simulink model "LW_ctrl"  (R2024b)
settings: Solver=ode4  StartTime=0.0  StopTime=SIM_TIME  FixedStep=0.001  RelTol=1e-3  EnableMultiTasking=on
StartFcn:
  | %timestart = cputime;
StopFcn:
  | %dt = cputime - timestart
undefined symbols (not defined in the file or in its folder): AttCtrl_cycle, ControlMode, DEG2RAD, Earth, FlightMode, LW_ACRO_P_MAX, LW_ACRO_R_MAX, LW_ACRO_Y_MAX, LW_AERO_C0, LW_AERO_C1, LW_AERO_Y0, LW_ANGLE, LW_DMZ0, LW_DMZ_MIN, LW_LAT_CIRCLE, LW_MAN_PITCH_MAX, LW_MAN_ROLL_MAX, LW_MASS, LW_OB_CIRCLE_R, LW_OB_CIRCLE_V, LW_OB_CIRCLE_W, LW_OB_TYPE, LW_REX_YAW, LW_SERVOL_MAX, LW_SERVOR_MAX, LW_THR_HOVER, LW_WZ_MAX, LW_X_ACCEL_MAX, LW_X_ACCEL_MIN, LW_X_FF, LW_X_JERK_MAX, LW_X_P, LW_X_VEL_MAX, LW_Y_ACCEL_MAX, LW_Y_ACCEL_MIN, LW_Y_FF, LW_Y_JERK_MAX, LW_Y_P, LW_Y_VEL_MAX, LW_YAW_KAD, LW_YAW_KAP, LW_Z_ACCEL_LOW, LW_Z_ACCEL_UP, LW_Z_FF, LW_Z_JERK_MAX, LW_Z_P, LW_Z_VEL_MAX_UP, Map_xoffset, Map_yoffset, Map_zoffset, MAX_wdotx, MAX_wdoty, MAX_wdotz, Mixer_cycle, ModelParam_AccelMax, ModelParam_DelayAtt, ModelParam_DelayOmega, ModelParam_DelayPos, ModelParam_envAltitude, ModelParam_envGravityAcc ... (+57)
libraries: pixhawk_slib_uORB_RW x15, simulink x6, slpidlib x6, dspstat3 x5, aerolibnav x4, aerolibtransform2 x3, pixhawk_slib_sensors_actuators x2, etargetslib x2, pixhawk_slib_rfly x1, aerolibatmos2 x1, slrealtimeiplib x1, SignalEditorBlockLib x1
(part 3 of 6)

== system LW_ctrl/Controller/PID_Controller/PID_Controller/toPWM ==
  T : Inport
  voltage : Inport  Port=2
  Bus Selector2 : BusSelector  OutputSignals=battery_status.voltage_filtered_v,battery_status.connected
  Constant : Constant  Value=single(1/ModelParam_rotorCt)
  Product : Product
  Sqrt : Sqrt
  toPWM : MATLAB Function  TreatAsAtomicUnit=on
  pwm : Outport  VectorParamsAs1DForOutWhenUnconnected=off
  wires:
  T/1 -> Product/1
  Product/1 -> Sqrt/1
  toPWM/1(pwm) -> pwm/1
  Constant/1 -> Product/2
  Sqrt/1 -> toPWM/1(w)
  voltage/1 -> Bus Selector2/1
  Bus Selector2/1 -> toPWM/2(voltage)  "<voltage_filtered_v>"
  Bus Selector2/2 -> toPWM/3(batt_connected)  "<connected>"

== system LW_ctrl/Output/OutputSelect/Sim/Lifting Body Airframe ==
  inPWM : Inport
  Constant : Constant  Value=SEND_TO_UNREAL
  Constant1 : Constant  Value=0
  Constant2 : Constant  Value=[0 0 0 0 0 0]  OutDataTypeStr=single
  Estimator : Subsystem
  Get Terrain : Subsystem
  Selector : Selector  InputPortWidth=8  IndexOptions=Index vector (dialog)  Indices=[1:6]  OutputSizes=1
  Subsystem Reference : Subsystem  ReferencedSubsystem=LW_noaileron_dynamic
  Switch : Switch  Criteria=u2 ~= 0  SaturateOnIntegerOverflow=off  InputSameDT=off
  Terminator : Terminator
  To Unreal : Subsystem  InitFcn=RflySim3D_config
  wires:
  inPWM/1 -> Selector/1
  Subsystem Reference/1 -> Estimator/1(vehicle_states), Get Terrain/1(vehicle_states), To Unreal/1(vehicle_states)  "vehicle_sates"
  Subsystem Reference/2 -> Estimator/2(environment_states)  "env_states"
  Subsystem Reference/3 -> Terminator/1
  Subsystem Reference/4 -> To Unreal/2(MotorRads)
  Get Terrain/1(z) -> Switch/1
  Constant/1 -> Switch/2
  Switch/1 -> Subsystem Reference/2
  Constant1/1 -> Switch/3
  Selector/1 -> Subsystem Reference/1  "pwm1~6"
  Constant2/1 -> Subsystem Reference/3

== system LW_ctrl/navigator/logger/HIL&FLY/get_delta_t ==
  timestamp : Inport
  Data Type Conversion : DataTypeConversion  OutDataTypeStr=single  SaturateOnIntegerOverflow=off  RndMeth=Floor
  Gain : Gain  Gain=1.0e-6
  Memory : Memory  InheritSampleTime=on
  Saturation : Saturate  UpperLimit=0.2  LowerLimit=0.001
  Sum : Sum  Inputs=|+-
  delta_t : Outport  VectorParamsAs1DForOutWhenUnconnected=off
  wires:
  Gain/1 -> Saturation/1
  timestamp/1 -> Memory/1, Sum/1
  Memory/1 -> Sum/2
  Sum/1 -> Gain/1
  Data Type Conversion/1 -> delta_t/1
  Saturation/1 -> Data Type Conversion/1

== system LW_ctrl/navigator/navigator_offboard/task select/task select ==
  timestamp : Inport
  flight_mode : Inport  Port=2
  pos : Inport  Port=3
  vel : Inport  Port=4
  q : Inport  Port=5
  v_wind : Inport  Port=6
  CH8 : Inport  Port=7
  Bus Creator2 : BusCreator  Inputs=10  OutDataTypeStr=Bus: offboard_bus
      settings: InheritFromInputs=off
  df,coor,wind : MATLAB Function  TreatAsAtomicUnit=on
  task : MATLAB Function  TreatAsAtomicUnit=on
  task1 : Outport
  wires:
  df,coor,wind/3(acc_ref) -> Bus Creator2/3  "acc"
  df,coor,wind/10(OB_TASK) -> Bus Creator2/10
  task/4(euler_ref) -> df,coor,wind/4(euler_ref)
  task/7(dotpsi) -> df,coor,wind/7(dotpsi)
  task/5(dot3x) -> df,coor,wind/5(dot3x)
  df,coor,wind/1(pos_ref) -> Bus Creator2/1  "pos"
  Bus Creator2/1 -> task1/1
  df,coor,wind/9(dotwb_ref) -> Bus Creator2/9
  df,coor,wind/7(beta) -> Bus Creator2/7
  flight_mode/1 -> task/2(flight_mode)
  df,coor,wind/2(vel_ref) -> Bus Creator2/2  "vel"
  task/3(acc_ref) -> df,coor,wind/3("acc_ref ")
  task/1(pos_ref) -> df,coor,wind/1("pos_ref ")
  task/2(vel_ref) -> df,coor,wind/2("vel_ref ")
  task/6(yaw_ref) -> df,coor,wind/6(yaw_ref)
  df,coor,wind/5(f_d) -> Bus Creator2/5
  df,coor,wind/8(wb_ref) -> Bus Creator2/8
  q/1 -> task/5(q)
  df,coor,wind/6(alpha) -> Bus Creator2/6
  df,coor,wind/4(q_ref) -> Bus Creator2/4  "q"
  timestamp/1 -> task/1(timestamp)
  pos/1 -> task/3(pos)
  vel/1 -> task/4(vel)
  v_wind/1 -> df,coor,wind/8(v_wind)
  CH8/1 -> task/6(CH8)

== system LW_ctrl/rc_receive/manual_ctrl_in/HIL&FLY V1.13.3/logger ==
  Bus Selector : BusSelector  OutputSignals=x,y,r,z,AU5,AU6,AU7,AU8,RC_Lost
  Data Type Conversion : DataTypeConversion  Priority=10  OutDataTypeStr=double  SaturateOnIntegerOverflow=off  RndMeth=Floor
  Data Type Conversion{1..4} (4 alike) : DataTypeConversion  Priority=10  OutDataTypeStr=single  SaturateOnIntegerOverflow=off  RndMeth=Floor
  Data Type Conversion{5..7,9} (4 alike) : DataTypeConversion  Priority=10  OutDataTypeStr=uint32  SaturateOnIntegerOverflow=off  RndMeth=Floor
  Data Type Conversion8 : DataTypeConversion  Priority=10  OutDataTypeStr=boolean  SaturateOnIntegerOverflow=off  RndMeth=Floor
  get_delta_t : Subsystem
  hrt_timestamp : MATLAB Function  TreatAsAtomicUnit=on
  uORB Write Advanced : pixhawk_slib_uORB_RW/uORB Write Advanced  Ts=0  uORB_AdvtQueue=on  uORB_FieldEnabledArr="0  0  0  1  0  0  0  0  0  0  0"  uORB_Topic_str=0  uORB_Struct_DT="[1  1  1  1  1]"  BlockInputCount=5  uORB_StructParams="[\"voltage_v\",\"voltage_filtered_v\",\"current_a\",\"current_filtered_a\",\"remaining\"]"  uORB_PortSizes="[1  1  1  1]"  MsgSizeOf=0  MW_update=true
      settings: SourceProductName=uORB Read / Write Blocks
  wires:
  hrt_timestamp/1(ts) -> Data Type Conversion/1
  Data Type Conversion/1 -> uORB Write Advanced/1, get_delta_t/1(timestamp)
  get_delta_t/1(delta_t) -> uORB Write Advanced/2
  [log_man] -> Bus Selector/1  "log_man"
  Bus Selector/1 -> Data Type Conversion1/1  "<x>"
  Bus Selector/2 -> Data Type Conversion2/1  "<y>"
  Bus Selector/3 -> Data Type Conversion3/1  "<r>"
  Bus Selector/4 -> Data Type Conversion4/1  "<z>"
  Bus Selector/5 -> Data Type Conversion5/1  "<AU5>"
  Bus Selector/6 -> Data Type Conversion6/1  "<AU6>"
  Bus Selector/7 -> Data Type Conversion7/1  "<AU7>"
  Bus Selector/9 -> Data Type Conversion8/1  "<RC_Lost>"
  Data Type Conversion1/1 -> uORB Write Advanced/3
  Data Type Conversion2/1 -> uORB Write Advanced/4
  Data Type Conversion3/1 -> uORB Write Advanced/5
  Data Type Conversion4/1 -> uORB Write Advanced/6
  Data Type Conversion5/1 -> uORB Write Advanced/7
  Data Type Conversion6/1 -> uORB Write Advanced/8
  Data Type Conversion7/1 -> uORB Write Advanced/9
  Data Type Conversion8/1 -> uORB Write Advanced/11
  Bus Selector/8 -> Data Type Conversion9/1  "<AU8>"
  Data Type Conversion9/1 -> uORB Write Advanced/10

== system LW_ctrl/rc_receive/manual_ctrl_in/Sim/Simulate RC ==
  Bus Creator : BusCreator  Inputs=9
  CH1 : Constant  Value=1500  OutDataTypeStr=uint16
  CH2 : Constant  Value=1500  OutDataTypeStr=uint16
  CH3 : Constant  Value=1600  OutDataTypeStr=uint16
  CH4 : Constant  Value=1500  OutDataTypeStr=uint16
  CH5 : Constant  Value=1000  OutDataTypeStr=uint16
  CH6 : Constant  Value=1000  OutDataTypeStr=uint16  SampleTime=-1
  CH7 : Constant  Value=1000  OutDataTypeStr=uint16
  CH8 : Constant  Value=1000  OutDataTypeStr=uint16
  Data Type Conversion{,1..4} (5 alike) : DataTypeConversion  OutDataTypeStr=single  SaturateOnIntegerOverflow=off  RndMeth=Floor
  InputConditioning : Subsystem
  RC_LOST : Constant  Value=false  OutDataTypeStr=uint16
  manual_ctrl_in : Outport  VectorParamsAs1DForOutWhenUnconnected=off
  wires:
  CH7/1 -> Data Type Conversion3/1
  Data Type Conversion1/1 -> Bus Creator/6  "AU6"
  InputConditioning/1(x) -> Bus Creator/1  "x"
  Bus Creator/1 -> manual_ctrl_in/1
  CH1/1 -> InputConditioning/1("ch1 ")
  InputConditioning/3(r) -> Bus Creator/3  "r"
  CH4/1 -> InputConditioning/4(ch4)
  InputConditioning/4(z) -> Bus Creator/4  "z"
  InputConditioning/2(y) -> Bus Creator/2  "y"
  Data Type Conversion3/1 -> Bus Creator/7  "AU7"
  Data Type Conversion/1 -> Bus Creator/5  "AU5"
  Data Type Conversion2/1 -> Bus Creator/9  "RC_Lost"
  CH2/1 -> InputConditioning/2(ch2)
  CH5/1 -> Data Type Conversion/1
  RC_LOST/1 -> Data Type Conversion2/1
  CH3/1 -> InputConditioning/3(ch3)
  CH6/1 -> Data Type Conversion1/1
  Data Type Conversion4/1 -> Bus Creator/8  "AU8"
  CH8/1 -> Data Type Conversion4/1

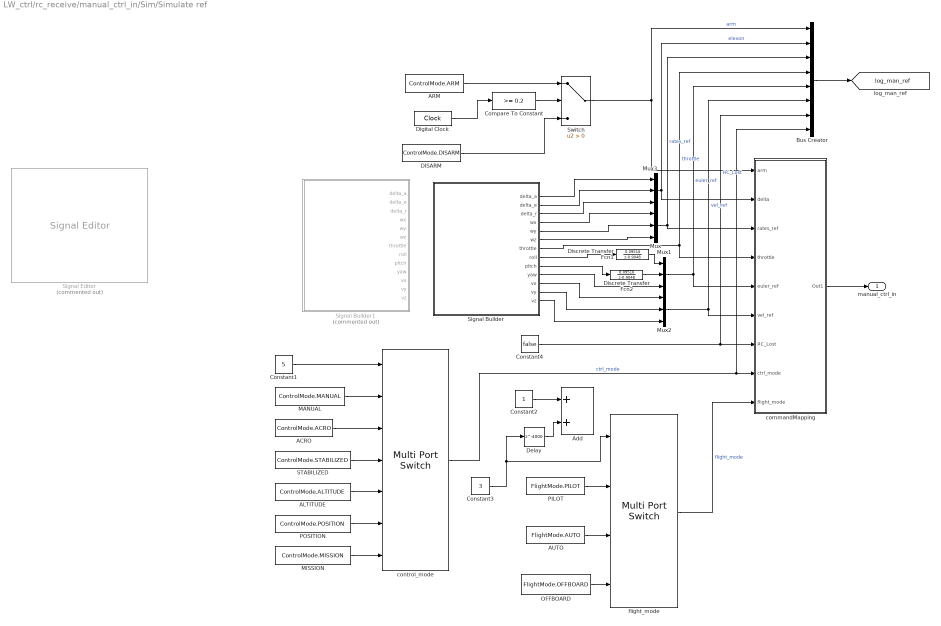
== system LW_ctrl/rc_receive/manual_ctrl_in/Sim/Simulate ref ==
  ACRO : Constant  Value=ControlMode.ACRO
  ALTITUDE : Constant  Value=ControlMode.ALTITUDE
  ARM : Constant  Value=ControlMode.ARM
  AUTO : Constant  Value=FlightMode.AUTO
  Add : Sum
  Bus Creator : BusCreator  Inputs=8
  Compare To Constant : simulink/Logic and Bit Operations/Compare To Constant  relop=>=  const=0.2  OutDataTypeStr=boolean
  Constant1 : Constant  Value=5
  Constant2 : Constant
  Constant3 : Constant  Value=3
  Constant4 : Constant  Value=false
  DISARM : Constant  Value=ControlMode.DISARM
  Delay : Delay  DelayLength=4000  InitialCondition=0
  Digital Clock : DigitalClock  SampleTime=-1
  Discrete Transfer Fcn1 : DiscreteTransferFcn  Numerator=0.09516  Denominator=[1 -0.9048]
  Discrete Transfer Fcn2 : DiscreteTransferFcn  Numerator=0.09516  Denominator=[1 -0.9048]
  MANUAL : Constant  Value=ControlMode.MANUAL
  MISSION : Constant  Value=ControlMode.MISSION
  Mux{,1..3} (4 alike) : Mux  Inputs=3
  OFFBOARD : Constant  Value=FlightMode.OFFBOARD
  PILOT : Constant  Value=FlightMode.PILOT
  POSITION : Constant  Value=ControlMode.POSITION
  STABILIZED : Constant  Value=ControlMode.STABILIZED
  Signal Builder : Subsystem  Tag=STV Subsys  LoadFcn=sigbuilder_block('load');  StartFcn=sigbuilder_block('start');  StopFcn=sigbuilder_block('stop');  ClipboardFcn=sigbuilder_block('clipboard');  TreatAsAtomicUnit=on  mask(Sigbuilder block){tuvar=[0:10]}
      mask help: Simulink:masks:SigbuilderBlock_MD
      mask init:
      | if ~strcmp(get_param(bdroot(gcbh),'SimulationStatus'),'stopped') tuvar = sigbuilder_block('maskInit'); end
      settings: CopyFcn=sigbuilder_block('copy');  DeleteFcn=sigbuilder_block('delete');  ModelCloseFcn=sigbuilder_block('modelClose');  PreSaveFcn=sigbuilder_block('preSave');  PauseFcn=sigbuilder_block('pause');  ContinueFcn=sigbuilder_block('continue');  NameChangeFcn=sigbuilder_block('namechange');  OpenFcn=sigbuilder_block('open',[16 10 1269 593 ]);  CloseFcn=sigbuilder_block('close');
      mask Display: plot(0, 0, 100, 100,[2, 2, 32, 32, 2], [68, 8, 8, 68, 68],[32, 2], [38, 38], [32, 19, 2],[53, 60, 44], [32, 17, 17, 2],[16, 16, 31, 31]);txt = getActiveGroup(gcbh);text(2, 100, txt,'verticalAlignment', 'top');
  Signal Builder1 : Subsystem  Tag=STV Subsys  Commented=on  LoadFcn=sigbuilder_block('load');  StartFcn=sigbuilder_block('start');  StopFcn=sigbuilder_block('stop');  ClipboardFcn=sigbuilder_block('clipboard');  TreatAsAtomicUnit=on  mask(Sigbuilder block){tuvar=[0:10]}
      mask help: Simulink:masks:SigbuilderBlock_MD
      mask init:
      | if ~strcmp(get_param(bdroot(gcbh),'SimulationStatus'),'stopped') tuvar = sigbuilder_block('maskInit'); end
      settings: CopyFcn=sigbuilder_block('copy');  DeleteFcn=sigbuilder_block('delete');  ModelCloseFcn=sigbuilder_block('modelClose');  PreSaveFcn=sigbuilder_block('preSave');  PauseFcn=sigbuilder_block('pause');  ContinueFcn=sigbuilder_block('continue');  NameChangeFcn=sigbuilder_block('namechange');  OpenFcn=sigbuilder_block('open',[0 0 1380.75 751.5 ]);  CloseFcn=sigbuilder_block('close');
      mask Display: plot(0, 0, 100, 100,[2, 2, 32, 32, 2], [68, 8, 8, 68, 68],[32, 2], [38, 38], [32, 19, 2],[53, 60, 44], [32, 17, 17, 2],[16, 16, 31, 31]);txt = getActiveGroup(gcbh);text(2, 100, txt,'verticalAlignment', 'top');
  Signal Editor : SignalEditorBlockLib/Signal Editor  Commented=on  FileName=simulation_ref.mat  ActiveScenario=Scenario  ActiveSignal=delta_a  IsBus=off  OutputBusObjectStr=Bus: BusObject  SampleTime=-1  Interpolate=off  ZeroCross=off  OutputAfterFinalValue=Holding final value  Unit=inherit  PreserveSignalName=on  ApplySigPropsToAllScenarios=on  ApplySigPropsToAllSignals=off
  Switch : Switch  Criteria=u2 > Threshold  SaturateOnIntegerOverflow=off  InputSameDT=off
  commandMapping : Subsystem
  control_mode : MultiPortSwitch  Inputs=6  SaturateOnIntegerOverflow=off  InputSameDT=off
  flight_mode : MultiPortSwitch  SaturateOnIntegerOverflow=off  InputSameDT=off
  manual_ctrl_in : Outport  VectorParamsAs1DForOutWhenUnconnected=off
  tag scope: log_man_ref=global
  wires:
  ALTITUDE/1 -> control_mode/5
  control_mode/1 -> Bus Creator/8, commandMapping/8(ctrl_mode)  "ctrl_mode"
  MISSION/1 -> control_mode/7
  Constant1/1 -> control_mode/1
  STABILIZED/1 -> control_mode/4
  ARM/1 -> Switch/1
  ACRO/1 -> control_mode/3
  DISARM/1 -> Switch/3
  POSITION/1 -> control_mode/6
  Switch/1 -> commandMapping/1(arm), Bus Creator/1  "arm"
  Constant4/1 -> Bus Creator/7, commandMapping/7(RC_Lost)  "RC_Lost"
  commandMapping/1(Out1) -> manual_ctrl_in/1
  Signal Builder/4(wx) -> Mux/1
  Signal Builder/5(wy) -> Mux/2
  Signal Builder/6(wz) -> Mux/3
  Mux/1 -> Bus Creator/3, commandMapping/3(rates_ref)  "rates_ref"
  Signal Builder/7(throttle) -> commandMapping/4(throttle), Bus Creator/4  "throttle"
  Signal Builder/8(roll) -> Discrete Transfer Fcn1/1
  Signal Builder/10(yaw) -> Mux1/3
  Mux1/1 -> Bus Creator/5, commandMapping/5(euler_ref)  "euler_ref"
  Mux2/1 -> Bus Creator/6, commandMapping/6(vel_ref)  "vel_ref"
  Bus Creator/1 -> [log_man_ref]
  Constant2/1 -> Add/1
  flight_mode/1 -> commandMapping/9(flight_mode)  "flight_mode"
  PILOT/1 -> flight_mode/2
  AUTO/1 -> flight_mode/3
  OFFBOARD/1 -> flight_mode/4
  Signal Builder/1(delta_a) -> Mux3/1
  Signal Builder/2(delta_e) -> Mux3/2
  Signal Builder/3(delta_r) -> Mux3/3
  Mux3/1 -> commandMapping/2(delta), Bus Creator/2  "elevon"
  MANUAL/1 -> control_mode/2
  Compare To Constant/1 -> Switch/2
  Digital Clock/1 -> Compare To Constant/1
  Discrete Transfer Fcn1/1 -> Mux1/1
  Signal Builder/9(pitch) -> Discrete Transfer Fcn2/1
  Discrete Transfer Fcn2/1 -> Mux1/2
  Constant3/1 -> flight_mode/1, Delay/1
  Delay/1 -> Add/2
  Signal Builder/12(vy) -> Mux2/2
  Signal Builder/13(vz) -> Mux2/3
  Signal Builder/11(vx) -> Mux2/1

== system LW_ctrl/rc_receive/manual_ctrl_in/Sim/joystick ==
  Bus Creator : BusCreator  Inputs=9
  Data Type Conversion{,1..6} (7 alike) : DataTypeConversion  OutDataTypeStr=single  SaturateOnIntegerOverflow=off  RndMeth=Floor
  Demux : Demux  Outputs=6
  MATLAB Function1 : MATLAB Function  TreatAsAtomicUnit=on
  Median Filter{,1..4} (5 alike) : dspstat3/Median Filter  WindowLength=5  SimulateUsing=Interpreted execution
  Pilot Joystick All : aerolibanimutils/Pilot Joystick  JoystickID=Joystick1  OutputConfiguration=AllOutputs  SampleTime=-1
  RC_LOST : Constant  Value=false  OutDataTypeStr=uint16
  Terminator1 : Terminator
  Terminator2 : Terminator
  Terminator3 : Terminator
  manual_ctrl_in : Outport  VectorParamsAs1DForOutWhenUnconnected=off
  wires:
  MATLAB Function1/7(AU7) -> Data Type Conversion3/1
  Data Type Conversion1/1 -> Bus Creator/6  "AU6"
  MATLAB Function1/1(x) -> Bus Creator/1  "x"
  Bus Creator/1 -> manual_ctrl_in/1
  MATLAB Function1/4(r) -> Bus Creator/3  "r"
  Demux/4 -> Median Filter4/1
  MATLAB Function1/3(z) -> Bus Creator/4  "z"
  MATLAB Function1/2(y) -> Bus Creator/2  "y"
  Data Type Conversion3/1 -> Bus Creator/7  "AU7"
  Data Type Conversion/1 -> Bus Creator/5  "AU5"
  Data Type Conversion2/1 -> Bus Creator/9  "RC_Lost"
  MATLAB Function1/5(AU5) -> Data Type Conversion/1
  MATLAB Function1/9(RC_LOST) -> Data Type Conversion2/1
  Demux/3 -> Median Filter3/1
  Pilot Joystick All/1 -> Data Type Conversion6/1
  Demux/6 -> Terminator1/1
  Pilot Joystick All/3 -> Terminator2/1
  Data Type Conversion4/1 -> Bus Creator/8  "AU8"
  MATLAB Function1/8(AU8) -> Data Type Conversion4/1
  Demux/1 -> Median Filter1/1
  Demux/2 -> Median Filter2/1
  MATLAB Function1/6(AU6) -> Data Type Conversion1/1  "arm"
  RC_LOST/1 -> MATLAB Function1/6(failsafe), MATLAB Function1/7(rc_lost)
  Pilot Joystick All/2 -> Data Type Conversion5/1
  Demux/5 -> Terminator3/1
  Median Filter/1 -> MATLAB Function1/5(states)
  Data Type Conversion5/1 -> Median Filter/1
  Median Filter1/1 -> MATLAB Function1/1(ch1)
  Median Filter2/1 -> MATLAB Function1/2(ch2)
  Median Filter3/1 -> MATLAB Function1/3(ch3)
  Median Filter4/1 -> MATLAB Function1/4(ch4)
  Data Type Conversion6/1 -> Demux/1

== system LW_ctrl/rc_receive/manual_ctrl_in/Sim/logger ==
  Bus Creator : BusCreator  Inputs=2
  log_manual_ctrl_in : ToFile  Filename=./log/SIM/log_manual_ctrl_in.mat  MatrixName=log_manual_ctrl_in  SaveFormat=Timeseries
  wires:
  Bus Creator/1 -> log_manual_ctrl_in/1  "log_man"
  [log_man_ref] -> Bus Creator/1  "log_man_ref"
  [log_man_rc] -> Bus Creator/2  "log_man_rc"

== system LW_ctrl/state_machine/logger/HIL&FLY/get_delta_t ==
  timestamp : Inport
  Data Type Conversion : DataTypeConversion  OutDataTypeStr=single  SaturateOnIntegerOverflow=off  RndMeth=Floor
  Gain : Gain  Gain=1.0e-6
  Memory : Memory  InheritSampleTime=on
  Saturation : Saturate  UpperLimit=0.2  LowerLimit=0.001
  Sum : Sum  Inputs=|+-
  delta_t : Outport  VectorParamsAs1DForOutWhenUnconnected=off
  wires:
  Gain/1 -> Saturation/1
  timestamp/1 -> Memory/1, Sum/1
  Memory/1 -> Sum/2
  Sum/1 -> Gain/1
  Data Type Conversion/1 -> delta_t/1
  Saturation/1 -> Data Type Conversion/1

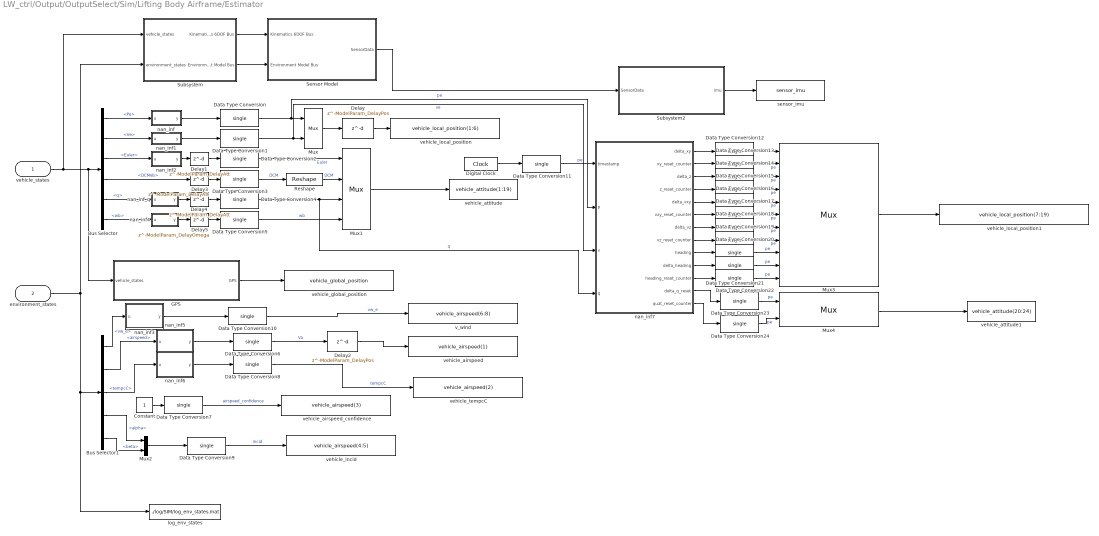
== system LW_ctrl/Output/OutputSelect/Sim/Lifting Body Airframe/Estimator ==
  vehicle_states : Inport
  environment_states : Inport  Port=2
  Bus Selector : BusSelector  OutputSignals=Pe,Ve,Euler,DCMeb,q,wb
  Bus Selector1 : BusSelector  OutputSignals=vw_e,airspeed,tempcC,alpha,beta
  Constant : Constant
  Data Type Conversion{,1..24} (25 alike) : DataTypeConversion  OutDataTypeStr=single  SaturateOnIntegerOverflow=off  RndMeth=Floor
  Delay : Delay  DelayLength=ModelParam_DelayPos  InitialCondition=0
  Delay1 : Delay  DelayLength=ModelParam_DelayAtt  InitialCondition=0
  Delay2 : Delay  DelayLength=ModelParam_DelayPos  InitialCondition=0
  Delay3 : Delay  DelayLength=ModelParam_DelayAtt  InitialCondition=0
  Delay4 : Delay  DelayLength=ModelParam_DelayAtt  InitialCondition=0
  Delay5 : Delay  DelayLength=ModelParam_DelayOmega  InitialCondition=0
  Digital Clock : DigitalClock  SampleTime=0.001
  GPS : Subsystem
  Mux : Mux  Inputs=2
      settings: DisplayOption=signals
  Mux1 : Mux
      settings: DisplayOption=signals
  Mux2 : Mux  Inputs=2
  Mux3 : Mux  Inputs=11
      settings: DisplayOption=signals
  Mux4 : Mux  Inputs=2
      settings: DisplayOption=signals
  Reshape : Reshape
  Sensor Model : Subsystem
  Subsystem : Subsystem
  Subsystem2 : Subsystem
  log_env_states : ToFile  Filename=./log/SIM/log_env_states.mat  MatrixName=log_env_states  SaveFormat=Timeseries
  nan_inf : MATLAB Function  TreatAsAtomicUnit=on
  nan_inf1 : MATLAB Function  TreatAsAtomicUnit=on
  nan_inf2 : MATLAB Function  TreatAsAtomicUnit=on
  nan_inf3 : MATLAB Function  TreatAsAtomicUnit=on
  nan_inf4 : MATLAB Function  TreatAsAtomicUnit=on
  nan_inf5 : MATLAB Function  TreatAsAtomicUnit=on
  nan_inf6 : MATLAB Function  TreatAsAtomicUnit=on
  nan_inf7 : MATLAB Function  TreatAsAtomicUnit=on
  nan_inf_q : MATLAB Function  TreatAsAtomicUnit=on
  sensor_imu : DataStoreWrite  DataStoreName=sensor_imu  IndexOptions=Index vector (dialog)  Indices=1  OutputSizes=1
  v_wind : DataStoreWrite  DataStoreName=vehicle_airspeed  DataStoreElements=vehicle_airspeed(6:8)  IndexOptions=Index vector (dialog)  Indices=1  OutputSizes=1
  vehicle_airspeed : DataStoreWrite  DataStoreName=vehicle_airspeed  DataStoreElements=vehicle_airspeed(1)  IndexOptions=Index vector (dialog)  Indices=1  OutputSizes=1
  vehicle_airspeed_confidence : DataStoreWrite  DataStoreName=vehicle_airspeed  DataStoreElements=vehicle_airspeed(3)  IndexOptions=Index vector (dialog)  Indices=1  OutputSizes=1
  vehicle_attitude : DataStoreWrite  DataStoreName=vehicle_attitude  DataStoreElements=vehicle_attitude(1:19)  IndexOptions=Index vector (dialog)  Indices=1  OutputSizes=1
  vehicle_attitude1 : DataStoreWrite  DataStoreName=vehicle_attitude  DataStoreElements=vehicle_attitude(20:24)  IndexOptions=Index vector (dialog)  Indices=1  OutputSizes=1
  vehicle_global_position : DataStoreWrite  DataStoreName=vehicle_global_position  IndexOptions=Index vector (dialog)  Indices=1  OutputSizes=1
  vehicle_incid : DataStoreWrite  DataStoreName=vehicle_airspeed  DataStoreElements=vehicle_airspeed(4:5)  IndexOptions=Index vector (dialog)  Indices=1  OutputSizes=1
  vehicle_local_position : DataStoreWrite  DataStoreName=vehicle_local_position  DataStoreElements=vehicle_local_position(1:6)  IndexOptions=Index vector (dialog)  Indices=1  OutputSizes=1
  vehicle_local_position1 : DataStoreWrite  DataStoreName=vehicle_local_position  DataStoreElements=vehicle_local_position(7:19)  IndexOptions=Index vector (dialog)  Indices=1  OutputSizes=1
  vehicle_tempcC : DataStoreWrite  DataStoreName=vehicle_airspeed  DataStoreElements=vehicle_airspeed(2)  IndexOptions=Index vector (dialog)  Indices=1  OutputSizes=1
  wires:
  vehicle_states/1 -> Subsystem/1(vehicle_states), GPS/1(vehicle_states), Bus Selector/1
  Bus Selector/1 -> nan_inf/1(u)  "<Pe>"
  Bus Selector/2 -> nan_inf1/1(u)  "<Ve>"
  Bus Selector/6 -> nan_inf4/1(u)  "<wb>"
  Bus Selector/4 -> Delay3/1  "<DCMeb>"
  Bus Selector/3 -> nan_inf2/1(u)  "<Euler>"
  Bus Selector/5 -> nan_inf_q/1(u)  "<q>"
  Constant/1 -> Data Type Conversion7/1
  Data Type Conversion/1 -> nan_inf7/2(p), Mux/1  "pe"
  Data Type Conversion1/1 -> nan_inf7/3(v), Mux/2  "ve"
  Data Type Conversion2/1 -> Mux1/1  "Euler"
  Reshape/1 -> Mux1/2  "DCM"
  Data Type Conversion4/1 -> nan_inf7/4(q), Mux1/3  "q"
  Data Type Conversion5/1 -> Mux1/4  "wb"
  Data Type Conversion6/1 -> Delay2/1  "Va"
  Data Type Conversion7/1 -> vehicle_airspeed_confidence/1  "airspeed_confidence"
  Mux/1 -> Delay/1
  Data Type Conversion3/1 -> Reshape/1  "DCM"
  Bus Selector1/3 -> nan_inf6/1(u)  "<tempcC>"
  Data Type Conversion8/1 -> vehicle_tempcC/1  "tempcC"
  Bus Selector1/2 -> nan_inf5/1(u)  "<airspeed>"
  nan_inf/1(y) -> Data Type Conversion/1
  nan_inf1/1(y) -> Data Type Conversion1/1
  nan_inf2/1(y) -> Delay1/1
  nan_inf_q/1(y) -> Delay4/1
  nan_inf4/1(y) -> Delay5/1
  nan_inf5/1(y) -> Data Type Conversion6/1
  nan_inf6/1(y) -> Data Type Conversion8/1
  Subsystem/1(Kinematics 6DOF Bus) -> Sensor Model/1(Kinematics 6DOF Bus)
  Subsystem/2(Environment Model Bus) -> Sensor Model/2(Environment Model Bus)
  Sensor Model/1(SensorData) -> Subsystem2/1(SensorData)
  environment_states/1 -> log_env_states/1, Bus Selector1/1, Subsystem/2(environment_states)
  GPS/1(GPS) -> vehicle_global_position/1
  Bus Selector1/4 -> Mux2/1  "<alpha>"
  Bus Selector1/5 -> Mux2/2  "<beta>"
  Mux2/1 -> Data Type Conversion9/1
  Data Type Conversion9/1 -> vehicle_incid/1  "incid"
  Delay/1 -> vehicle_local_position/1
  Mux1/1 -> vehicle_attitude/1
  Delay2/1 -> vehicle_airspeed/1
  Delay1/1 -> Data Type Conversion2/1
  Delay3/1 -> Data Type Conversion3/1
  Delay4/1 -> Data Type Conversion4/1
  Delay5/1 -> Data Type Conversion5/1
  Bus Selector1/1 -> nan_inf3/1(u)  "<vw_e>"
  nan_inf3/1(y) -> Data Type Conversion10/1
  Data Type Conversion10/1 -> v_wind/1  "vw_e"
  Subsystem2/1(imu) -> sensor_imu/1
  nan_inf7/1(delta_xy) -> Data Type Conversion12/1
  nan_inf7/2(xy_reset_counter) -> Data Type Conversion13/1
  nan_inf7/3(delta_z) -> Data Type Conversion14/1
  nan_inf7/4(z_reset_counter) -> Data Type Conversion15/1
  nan_inf7/5(delta_vxy) -> Data Type Conversion16/1
  nan_inf7/6(vxy_reset_counter) -> Data Type Conversion17/1
  nan_inf7/7(delta_vz) -> Data Type Conversion18/1
  nan_inf7/8(vz_reset_counter) -> Data Type Conversion19/1
  nan_inf7/9(heading) -> Data Type Conversion20/1
  nan_inf7/10(delta_heading) -> Data Type Conversion21/1
  nan_inf7/11(heading_reset_counter) -> Data Type Conversion22/1
  Mux3/1 -> vehicle_local_position1/1
  Digital Clock/1 -> Data Type Conversion11/1
  nan_inf7/12(delta_q_reset) -> Data Type Conversion23/1
  nan_inf7/13(quat_reset_counter) -> Data Type Conversion24/1
  Mux4/1 -> vehicle_attitude1/1
  Data Type Conversion11/1 -> nan_inf7/1(timestamp)  "pe"
  Data Type Conversion12/1 -> Mux3/1
  Data Type Conversion13/1 -> Mux3/2  "pe"
  Data Type Conversion14/1 -> Mux3/3  "pe"
  Data Type Conversion15/1 -> Mux3/4  "pe"
  Data Type Conversion16/1 -> Mux3/5  "pe"
  Data Type Conversion17/1 -> Mux3/6  "pe"
  Data Type Conversion18/1 -> Mux3/7  "pe"
  Data Type Conversion19/1 -> Mux3/8  "pe"
  Data Type Conversion20/1 -> Mux3/9  "pe"
  Data Type Conversion21/1 -> Mux3/10  "pe"
  Data Type Conversion22/1 -> Mux3/11  "pe"
  Data Type Conversion24/1 -> Mux4/2  "pe"
  Data Type Conversion23/1 -> Mux4/1  "pe"

== system LW_ctrl/Output/OutputSelect/Sim/Lifting Body Airframe/Get Terrain ==
  vehicle_states : Inport
  Bus Selector : BusSelector  OutputSignals=Pe
  Demux : Demux  Outputs=3
  Terminator : Terminator
  getTerrainAltData : MATLAB Function  TreatAsAtomicUnit=on
  z : Outport
  wires:
  Demux/3 -> Terminator/1
  Bus Selector/1 -> Demux/1  "<Pe>"
  Demux/2 -> getTerrainAltData/2(y)
  Demux/1 -> getTerrainAltData/1(x)
  getTerrainAltData/1(z) -> z/1
  vehicle_states/1 -> Bus Selector/1

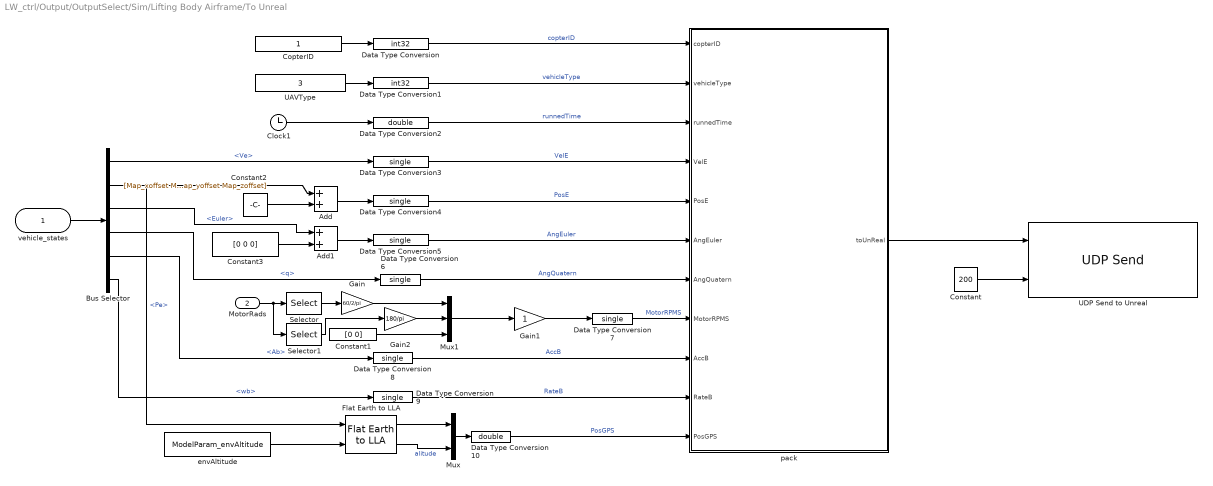
== system LW_ctrl/Output/OutputSelect/Sim/Lifting Body Airframe/To Unreal ==
  vehicle_states : Inport
  MotorRads : Inport  Port=2
  Add : Sum
  Add1 : Sum
  Bus Selector : BusSelector  OutputSignals=Ve,Pe,Euler,q,Ab,wb
  Clock1 : Clock
  Constant : Constant  Value=200
  Constant1 : Constant  Value=[0 0]
  Constant2 : Constant  Value=[Map_xoffset Map_yoffset Map_zoffset]
  Constant3 : Constant  Value=[0 0 0]
  CopterID : Constant
  Data Type Conversion : DataTypeConversion  OutDataTypeStr=int32  SaturateOnIntegerOverflow=off  RndMeth=Floor
  Data Type Conversion1 : DataTypeConversion  OutDataTypeStr=int32  SaturateOnIntegerOverflow=off  RndMeth=Floor
  Data Type Conversion10 : DataTypeConversion  OutDataTypeStr=double  SaturateOnIntegerOverflow=off  RndMeth=Floor
  Data Type Conversion2 : DataTypeConversion  OutDataTypeStr=double  SaturateOnIntegerOverflow=off  RndMeth=Floor
  Data Type Conversion{3..9} (7 alike) : DataTypeConversion  OutDataTypeStr=single  SaturateOnIntegerOverflow=off  RndMeth=Floor
  Flat Earth to LLA : aerolibtransform2/Flat Earth to LLA  units=Metric (MKS)  ptype=Earth (WGS84)  F=1/298.257223563  R=6378137  refPosPort=off  LL0=ModelParam_GPSLatLong  psi=0
  Gain : Gain  Gain=60/2/pi
  Gain1 : Gain
  Gain2 : Gain  Gain=180/pi
  Mux : Mux  Inputs=2
  Mux1 : Mux  Inputs=3
  Selector : Selector  InputPortWidth=6  IndexOptions=Index vector (dialog)  Indices=[1:4]  OutputSizes=1
  Selector1 : Selector  InputPortWidth=6  IndexOptions=Index vector (dialog)  Indices=[5:6]  OutputSizes=1
  UAVType : Constant  Value=3
  "UDP Send to Unreal " : slrealtimeiplib/UDP Send  useHostTargetConn=on  toAddress='127.0.0.1'  toPort=20010  sampleTime=SampleTime  enableMessage=off  ipAddress=10.10.10.15  localPort=38820
  envAltitude : Constant  Value=ModelParam_envAltitude
  pack : Subsystem
  wires:
  pack/1(toUnReal) -> "UDP Send to Unreal "/1
  Constant/1 -> "UDP Send to Unreal "/2
  UAVType/1 -> Data Type Conversion1/1
  Data Type Conversion5/1 -> pack/6(AngEuler)  "AngEuler"
  Data Type Conversion7/1 -> pack/8(MotorRPMS)  "MotorRPMS"
  Clock1/1 -> Data Type Conversion2/1
  Data Type Conversion10/1 -> pack/11(PosGPS)  "PosGPS"
  Data Type Conversion9/1 -> pack/10(RateB)  "RateB"
  Data Type Conversion3/1 -> pack/4("VelE ")  "VelE"
  Data Type Conversion2/1 -> pack/3(runnedTime)  "runnedTime"
  Data Type Conversion8/1 -> pack/9(AccB)  "AccB"
  Bus Selector/3 -> Add1/1  "<Euler>"
  Data Type Conversion/1 -> pack/1(copterID)  "copterID"
  Data Type Conversion1/1 -> pack/2(vehicleType)  "vehicleType"
  CopterID/1 -> Data Type Conversion/1
  Bus Selector/1 -> Data Type Conversion3/1  "<Ve>"
  Bus Selector/4 -> Data Type Conversion6/1  "<q>"
  MotorRads/1 -> Selector1/1, Selector/1
  Bus Selector/5 -> Data Type Conversion8/1  "<Ab>"
  Data Type Conversion4/1 -> pack/5(PosE)  "PosE"
  Mux1/1 -> Gain1/1
  Bus Selector/6 -> Data Type Conversion9/1  "<wb>"
  Data Type Conversion6/1 -> pack/7(AngQuatern)  "AngQuatern"
  Mux/1 -> Data Type Conversion10/1
  vehicle_states/1 -> Bus Selector/1
  envAltitude/1 -> Flat Earth to LLA/2
  Bus Selector/2 -> Add/1, Flat Earth to LLA/1  "<Pe>"
  Flat Earth to LLA/1 -> Mux/1
  Flat Earth to LLA/2 -> Mux/2  "alitude"
  Gain/1 -> Mux1/1
  Constant1/1 -> Mux1/3
  Gain1/1 -> Data Type Conversion7/1
  Gain2/1 -> Mux1/2
  Selector/1 -> Gain/1
  Selector1/1 -> Gain2/1
  Add/1 -> Data Type Conversion4/1
  Constant2/1 -> Add/2
  Add1/1 -> Data Type Conversion5/1
  Constant3/1 -> Add1/2

== system LW_ctrl/rc_receive/manual_ctrl_in/HIL&FLY V1.13.3/logger/get_delta_t ==
  timestamp : Inport
  Data Type Conversion : DataTypeConversion  OutDataTypeStr=single  SaturateOnIntegerOverflow=off  RndMeth=Floor
  Gain : Gain  Gain=1.0e-6
  Memory : Memory  InheritSampleTime=on
  Saturation : Saturate  UpperLimit=0.2  LowerLimit=0.001
  Sum : Sum  Inputs=|+-
  delta_t : Outport  VectorParamsAs1DForOutWhenUnconnected=off
  wires:
  Gain/1 -> Saturation/1
  timestamp/1 -> Memory/1, Sum/1
  Memory/1 -> Sum/2
  Sum/1 -> Gain/1
  Data Type Conversion/1 -> delta_t/1
  Saturation/1 -> Data Type Conversion/1

== system LW_ctrl/rc_receive/manual_ctrl_in/Sim/Simulate RC/InputConditioning ==
  "ch1 " : Inport
  ch2 : Inport  Port=2
  ch3 : Inport  Port=3
  ch4 : Inport  Port=4
  Data Type Conversion{,1..3} (4 alike) : DataTypeConversion  OutDataTypeStr=single  SaturateOnIntegerOverflow=off  RndMeth=Floor
  Saturation{1..3,9} (4 alike) : Saturate  UpperLimit=1  LowerLimit=-1
  deadzone0 : MATLAB Function  TreatAsAtomicUnit=on
  deadzone1 : MATLAB Function  TreatAsAtomicUnit=on
  deadzone2 : MATLAB Function  TreatAsAtomicUnit=on
  deadzone3 : MATLAB Function  TreatAsAtomicUnit=on
  rc1_max : Constant  Value=RC1_MAX
  rc1_min : Constant  Value=RC1_MIN
  rc2_max : Constant  Value=RC2_MAX
  rc2_min : Constant  Value=RC2_MIN
  rc3_max : Constant  Value=RC3_MAX
  rc3_min : Constant  Value=RC3_MIN
  rc4_max : Constant  Value=RC4_MAX
  rc4_min : Constant  Value=RC4_MIN
  x : Outport  VectorParamsAs1DForOutWhenUnconnected=off
  y : Outport  Port=2  VectorParamsAs1DForOutWhenUnconnected=off
  r : Outport  Port=3  VectorParamsAs1DForOutWhenUnconnected=off
  z : Outport  Port=4  VectorParamsAs1DForOutWhenUnconnected=off
  wires:
  Saturation9/1 -> y/1
  "ch1 "/1 -> Data Type Conversion/1
  deadzone0/1(y) -> Saturation9/1
  deadzone3/1(y) -> Saturation3/1
  rc1_min/1 -> deadzone0/2(rc_min)
  rc1_max/1 -> deadzone0/3(rc_max)
  Data Type Conversion/1 -> deadzone0/1(u)
  Data Type Conversion1/1 -> deadzone1/1(u)
  rc2_max/1 -> deadzone1/3(rc_max)
  rc2_min/1 -> deadzone1/2(rc_min)
  deadzone1/1(y) -> Saturation1/1
  ch2/1 -> Data Type Conversion1/1
  Saturation1/1 -> x/1
  Data Type Conversion2/1 -> deadzone2/1(u)
  rc4_max/1 -> deadzone2/3(rc_max)
  rc4_min/1 -> deadzone2/2(rc_min)
  deadzone2/1(y) -> Saturation2/1
  ch4/1 -> Data Type Conversion2/1
  Saturation2/1 -> r/1
  ch3/1 -> Data Type Conversion3/1
  rc3_min/1 -> deadzone3/2(rc_min)
  rc3_max/1 -> deadzone3/3(rc_max)
  Data Type Conversion3/1 -> deadzone3/1(u)
  Saturation3/1 -> z/1

== system LW_ctrl/rc_receive/manual_ctrl_in/Sim/Simulate ref/Signal Builder ==
  Demux : Demux  Tag=STV Demux  Outputs=13
      settings: DisplayOption=none
  FromWs : FromWorkspace  Tag=STV FromWs  VariableName=tuvar  SampleTime=-1
      SigBuilderData=|
      | common.afterFinalStr = 'Extrapolate'
      | common.sampleTime = 0
      | dataSet.timeRange = [0 100]
      | dataSet.name = 'Group 1'
      | sbobj.Groups.Name = 'Group 1'
      | sbobj.Groups.Signals(1).Name = 'delta_a'
      | sbobj.Groups.Signals(1).XData = [0 4 5 15 20 100]
      | sbobj.Groups.Signals(1).YData = [0 0 60 60 0 0]
      | sbobj.Groups.Signals(2).Name = 'delta_e'
      | sbobj.Groups.Signals(2).XData = [0 5 8 15 20 100]
      | sbobj.Groups.Signals(2).YData = [0 0 0 0 0 0]
      | sbobj.Groups.Signals(3).Name = 'delta_r'
      | sbobj.Groups.Signals(3).XData = [0 4 5 6 8 100]
      | sbobj.Groups.Signals(3).YData = [0 0 0 0 0 0]
      | sbobj.Groups.Signals(4).Name = 'wx'
      | sbobj.Groups.Signals(4).XData = [0 4 5 6 8 100]
      | sbobj.Groups.Signals(4).YData = [0 0 10 10 0 0]
      | sbobj.Groups.Signals(5).Name = 'wy'
      | sbobj.Groups.Signals(5).XData = [0 50 60 70 80 100]
      | sbobj.Groups.Signals(5).YData = [0 0 20 20 0 0]
      | sbobj.Groups.Signals(6).Name = 'wz'
      | sbobj.Groups.Signals(6).XData = [0 1 4 8 11 65.7 72.6 100]
      | sbobj.Groups.Signals(6).YData = [0 0 0 0 0 0 0 0]
      | sbobj.Groups.Signals(7).Name = 'throttle'
      | sbobj.Groups.Signals(7).XData = [0 1 5 6 8 35.9 36 37 100]
      | sbobj.Groups.Signals(7).YData = [0 0.55 0.6 0.5 0.5 0.5 0 0.1 0.3]
      | sbobj.Groups.Signals(8).Name = 'roll'
      | sbobj.Groups.Signals(8).XData = [0 48 50 55 58 100]
      | sbobj.Groups.Signals(8).YData = [0 0 10 10 0 0]
      | sbobj.Groups.Signals(9).Name = 'pitch'
      | sbobj.Groups.Signals(9).XData = [0 15 40 45 60.3 68.8 100]
      | sbobj.Groups.Signals(9).YData = [0 0 0 -25 -25 0 0]
      | sbobj.Groups.Signals(10).Name = 'yaw'
      | sbobj.Groups.Signals(10).XData = [0 25 26 29 30 100]
      | sbobj.Groups.Signals(10).YData = [0 0 0 0 0 0]
      | sbobj.Groups.Signals(11).Name = 'vx'
      | sbobj.Groups.Signals(11).XData = [0 8 40 40.3 55 60 100]
      | sbobj.Groups.Signals(11).YData = [0 0 0 0 0 0 0]
      | sbobj.Groups.Signals(12).Name = 'vy'
      | sbobj.Groups.Signals(12).XData = [0 50 53 56 80 85 90 100]
      | sbobj.Groups.Signals(12).YData = [0 0 0 0 0 0 0 0]
      | sbobj.Groups.Signals(13).Name = 'vz'
      | sbobj.Groups.Signals(13).XData = [0 1 2 10 12 95 100]
      | sbobj.Groups.Signals(13).YData = [0 0 -3 -3 0 0 0]
      | sbobj.Groups.TimeRange = [0 100]
  delta_a : Outport  Tag=STV Outport
  delta_e : Outport  Tag=STV Outport  Port=2
  delta_r : Outport  Tag=STV Outport  Port=3
  wx : Outport  Tag=STV Outport  Port=4
  wy : Outport  Tag=STV Outport  Port=5
  wz : Outport  Tag=STV Outport  Port=6
  throttle : Outport  Tag=STV Outport  Port=7
  roll : Outport  Tag=STV Outport  Port=8
  pitch : Outport  Tag=STV Outport  Port=9
  yaw : Outport  Tag=STV Outport  Port=10
  vx : Outport  Tag=STV Outport  Port=11
  vy : Outport  Tag=STV Outport  Port=12
  vz : Outport  Tag=STV Outport  Port=13
  wires:
  FromWs/1 -> Demux/1
  Demux/1 -> delta_a/1
  Demux/2 -> delta_e/1
  Demux/3 -> delta_r/1
  Demux/4 -> wx/1
  Demux/5 -> wy/1
  Demux/6 -> wz/1
  Demux/7 -> throttle/1
  Demux/8 -> roll/1
  Demux/9 -> pitch/1
  Demux/10 -> yaw/1
  Demux/11 -> vx/1
  Demux/12 -> vy/1
  Demux/13 -> vz/1

== system LW_ctrl/rc_receive/manual_ctrl_in/Sim/Simulate ref/Signal Builder1 ==
  Demux : Demux  Tag=STV Demux  Outputs=13
      settings: DisplayOption=none
  FromWs : FromWorkspace  Tag=STV FromWs  VariableName=tuvar  SampleTime=-1
      SigBuilderData=|
      | common.afterFinalStr = 'Extrapolate'
      | common.sampleTime = 0
      | dataSet.timeRange = [0 100]
      | dataSet.name = 'Group 1'
      | sbobj.Groups.Name = 'Group 1'
      | sbobj.Groups.Signals(1).Name = 'delta_a'
      | sbobj.Groups.Signals(1).XData = [0 4 5 15 20 100]
      | sbobj.Groups.Signals(1).YData = [0 0 60 60 0 0]
      | sbobj.Groups.Signals(2).Name = 'delta_e'
      | sbobj.Groups.Signals(2).XData = [0 5 8 15 20 100]
      | sbobj.Groups.Signals(2).YData = [0 0 0 0 0 0]
      | sbobj.Groups.Signals(3).Name = 'delta_r'
      | sbobj.Groups.Signals(3).XData = [0 4 5 6 8 100]
      | sbobj.Groups.Signals(3).YData = [0 0 0 0 0 0]
      | sbobj.Groups.Signals(4).Name = 'wx'
      | sbobj.Groups.Signals(4).XData = [0 4 5 6 8 100]
      | sbobj.Groups.Signals(4).YData = [0 0 0 0 0 0]
      | sbobj.Groups.Signals(5).Name = 'wy'
      | sbobj.Groups.Signals(5).XData = [0 50 60 70 80 100]
      | sbobj.Groups.Signals(5).YData = [0 0 0 0 0 0]
      | sbobj.Groups.Signals(6).Name = 'wz'
      | sbobj.Groups.Signals(6).XData = [0 50 60 70 80 100]
      | sbobj.Groups.Signals(6).YData = [0 0 0 0 0 0]
      | sbobj.Groups.Signals(7).Name = 'throttle'
      | sbobj.Groups.Signals(7).XData = [0 1 5 6 8 100]
      | sbobj.Groups.Signals(7).YData = [0 0.7 0.7 0.5 0.5 0.5]
      | sbobj.Groups.Signals(8).Name = 'roll'
      | sbobj.Groups.Signals(8).XData = [0 20 21 22 60 61 62 100]
      | sbobj.Groups.Signals(8).YData = [0 0 10 0 0 -10 0 0]
      | sbobj.Groups.Signals(9).Name = 'pitch'
      | sbobj.Groups.Signals(9).XData = [0 15 15 30 30.3 48.8 49.2 100]
      | sbobj.Groups.Signals(9).YData = [0 0 -30 -30 0 0 0 0]
      | sbobj.Groups.Signals(10).Name = 'yaw'
      | sbobj.Groups.Signals(10).XData = [0 25 26 29 30 100]
      | sbobj.Groups.Signals(10).YData = [0 0 0 0 0 0]
      | sbobj.Groups.Signals(11).Name = 'vx'
      | sbobj.Groups.Signals(11).XData = [0 8 30 40 60 70 90 100]
      | sbobj.Groups.Signals(11).YData = [0 0 0 20 20 0 0 0]
      | sbobj.Groups.Signals(12).Name = 'vy'
      | sbobj.Groups.Signals(12).XData = [0 45 50 55 80 85 90 100]
      | sbobj.Groups.Signals(12).YData = [0 0 -10 0 0 10 0 0]
      | sbobj.Groups.Signals(13).Name = 'vz'
      | sbobj.Groups.Signals(13).XData = [0 1 2 9 10 25 100]
      | sbobj.Groups.Signals(13).YData = [0 0 -1 -1 0 0 0]
      | sbobj.Groups.TimeRange = [0 100]
  delta_a : Outport  Tag=STV Outport
  delta_e : Outport  Tag=STV Outport  Port=2
  delta_r : Outport  Tag=STV Outport  Port=3
  wx : Outport  Tag=STV Outport  Port=4
  wy : Outport  Tag=STV Outport  Port=5
  wz : Outport  Tag=STV Outport  Port=6
  throttle : Outport  Tag=STV Outport  Port=7
  roll : Outport  Tag=STV Outport  Port=8
  pitch : Outport  Tag=STV Outport  Port=9
  yaw : Outport  Tag=STV Outport  Port=10
  vx : Outport  Tag=STV Outport  Port=11
  vy : Outport  Tag=STV Outport  Port=12
  vz : Outport  Tag=STV Outport  Port=13
  wires:
  Demux/13 -> vz/1
  Demux/12 -> vy/1
  Demux/11 -> vx/1
  Demux/10 -> yaw/1
  Demux/9 -> pitch/1
  Demux/8 -> roll/1
  Demux/7 -> throttle/1
  Demux/6 -> wz/1
  Demux/5 -> wy/1
  Demux/4 -> wx/1
  Demux/3 -> delta_r/1
  Demux/2 -> delta_e/1
  Demux/1 -> delta_a/1
  FromWs/1 -> Demux/1

== system LW_ctrl/rc_receive/manual_ctrl_in/Sim/Simulate ref/commandMapping ==
  arm : Inport
  delta : Inport  Port=2
  rates_ref : Inport  Port=3
  throttle : Inport  Port=4
  euler_ref : Inport  Port=5
  vel_ref : Inport  Port=6
  RC_Lost : Inport  Port=7
  ctrl_mode : Inport  Port=8
  flight_mode : Inport  Port=9
  Add : Sum
  Bus Creator : BusCreator  Inputs=9
  Compare To Constant : simulink/Logic and Bit Operations/Compare To Constant  relop===  const=ControlMode.ARM  OutDataTypeStr=boolean
  Constant : Constant  Value=1000
  Constant2 : Constant  Value=1000
  Constant3 : Constant  Value=0
  Data Type Conversion{,1..3} (4 alike) : DataTypeConversion  OutDataTypeStr=single  SaturateOnIntegerOverflow=off  RndMeth=Floor
  Demux : Demux  Outputs=6
  Gain1 : Gain  Gain=RC1_REV
  Gain2 : Gain  Gain=RC1_REV
  Gain3 : Gain  Gain=RC3_REV
  Gain4 : Gain  Gain=RC4_REV
  MATLAB Function : MATLAB Function  TreatAsAtomicUnit=on
  Switch : Switch  Criteria=u2 > Threshold  SaturateOnIntegerOverflow=off  InputSameDT=off
  command2pwm : Subsystem
  Out1 : Outport
  wires:
  Switch/1 -> Add/2
  Compare To Constant/1 -> Switch/2
  Constant2/1 -> Switch/1
  Demux/1 -> Gain1/1  "x"
  Data Type Conversion2/1 -> command2pwm/3(euler_ref)
  Data Type Conversion1/1 -> command2pwm/5(throttle)
  command2pwm/1(manual_ref) -> Demux/1
  Demux/6 -> Bus Creator/7  "AU7"
  Data Type Conversion/1 -> command2pwm/1(rates_ref)
  Demux/5 -> Bus Creator/5  "AU5"
  Demux/2 -> Gain2/1  "y"
  Data Type Conversion3/1 -> command2pwm/4(vel_ref)
  Constant/1 -> Add/1
  Demux/4 -> Gain4/1  "r"
  Demux/3 -> Gain3/1  "z"
  Constant3/1 -> Switch/3
  Add/1 -> Bus Creator/6  "AU6"
  Bus Creator/1 -> Out1/1
  vel_ref/1 -> Data Type Conversion3/1
  ctrl_mode/1 -> command2pwm/2(ctrl_mode)
  euler_ref/1 -> Data Type Conversion2/1
  RC_Lost/1 -> Bus Creator/9
  arm/1 -> Compare To Constant/1
  throttle/1 -> Data Type Conversion1/1
  rates_ref/1 -> Data Type Conversion/1
  flight_mode/1 -> MATLAB Function/1(flight_mode)
  MATLAB Function/1(AU8) -> Bus Creator/8  "AU8"
  delta/1 -> command2pwm/6(delta)
  Gain2/1 -> Bus Creator/2  "y"
  Gain1/1 -> Bus Creator/1  "x"
  Gain3/1 -> Bus Creator/3  "z"
  Gain4/1 -> Bus Creator/4  "r"

== system LW_ctrl/Output/OutputSelect/Sim/Lifting Body Airframe/Estimator/GPS ==
  vehicle_states : Inport
  Bus Selector : BusSelector  OutputSignals=Pe,Ve,Euler
  Data Type Conversion : DataTypeConversion  OutDataTypeStr=single  SaturateOnIntegerOverflow=off  RndMeth=Floor
  Demux : Demux  Outputs=3
  Demux1 : Demux  Outputs=3
  Flat Earth to LLA : aerolibtransform2/Flat Earth to LLA  units=Metric (MKS)  ptype=Earth (WGS84)  F=1/298.257223563  R=6378137  refPosPort=off  LL0=ModelParam_GPSLatLong  psi=0
  Gain : Gain  Gain=1e7
  Gain2 : Gain  Gain=1e7
  Gain3 : Gain  Gain=1e3
  ModelParam.GPSEphFinal : Constant  Value=ModelParam_GPSEphFinal
  ModelParam.GPSEpvFinal : Constant  Value=ModelParam_GPSEpvFinal
  ModelParam_envAltitude : Constant  Value=ModelParam_envAltitude
  Mux : Mux  Inputs=2
  Mux1 : Mux  Inputs=15
  Saturation : Saturate  UpperLimit=100000  LowerLimit=0
  alt_reset_counter : Constant  Value=0
  courseAngle : MATLAB Function  TreatAsAtomicUnit=on
  dead_reckoning : Constant  Value=0
  delta_alt : Constant  Value=0
  lat_lon_reset_counter : Constant  Value=0
  terrain_alt : Constant  Value=0
  terrain_alt_valid : Constant  Value=0
  GPS : Outport
  wires:
  Saturation/1 -> Mux/2
  lat_lon_reset_counter/1 -> Mux1/5  "lat_lon_reset_counter"
  delta_alt/1 -> Mux1/4  "delta_alt"
  courseAngle/1(course_angle) -> Mux1/10  "yaw"
  Demux1/3 -> Mux1/9  "vd"
  Demux1/2 -> Mux1/8  "ve"
  Demux1/1 -> Mux1/7  "vn"
  Mux1/1 -> Data Type Conversion/1
  ModelParam.GPSEpvFinal/1 -> Mux1/12  "epv"
  ModelParam.GPSEphFinal/1 -> Mux1/11  "eph"
  Demux/3 -> Gain3/1  "alt"
  Demux/1 -> Gain/1  "lat"
  Demux/2 -> Gain2/1  "lon"
  Mux/1 -> Demux/1
  Flat Earth to LLA/2 -> Saturation/1
  Flat Earth to LLA/1 -> Mux/1
  ModelParam_envAltitude/1 -> Flat Earth to LLA/2
  alt_reset_counter/1 -> Mux1/6  "alt_reset_counter"
  terrain_alt/1 -> Mux1/13  "terrain_alt"
  terrain_alt_valid/1 -> Mux1/14  "terrain_alt_valid"
  dead_reckoning/1 -> Mux1/15  "terrain_alt_valid"
  vehicle_states/1 -> Bus Selector/1
  Bus Selector/1 -> Flat Earth to LLA/1  "<Pe>"
  Bus Selector/2 -> Demux1/1, courseAngle/1(v)  "<Ve>"
  Gain/1 -> Mux1/1  "lat"
  Gain2/1 -> Mux1/2  "lon"
  Gain3/1 -> Mux1/3  "lon"
  Data Type Conversion/1 -> GPS/1
  Bus Selector/3 -> courseAngle/2(euler)  "<Euler>"

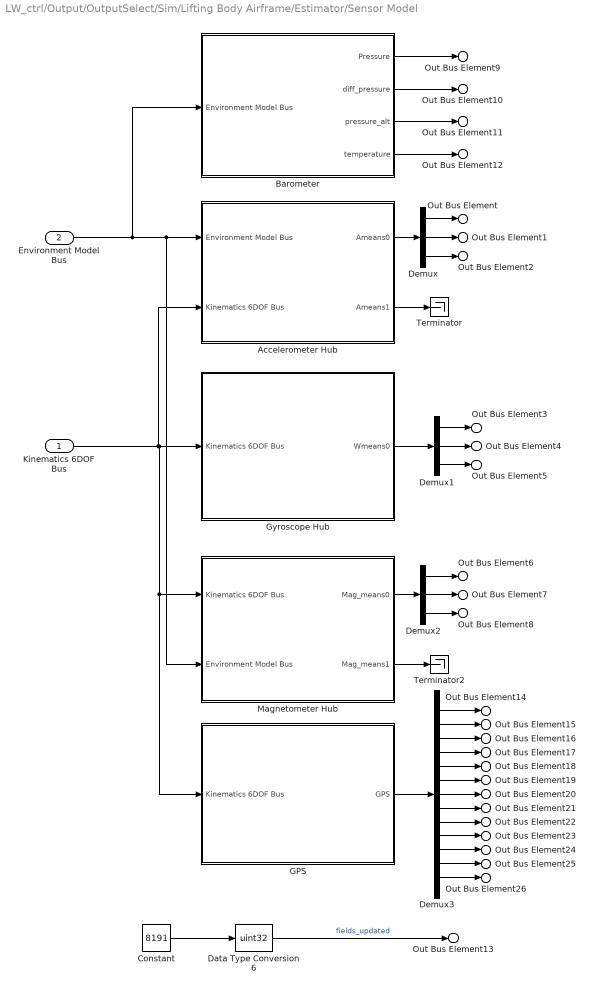
== system LW_ctrl/Output/OutputSelect/Sim/Lifting Body Airframe/Estimator/Sensor Model ==
  Kinematics 6DOF Bus : Inport
  Environment Model Bus : Inport  Port=2
  Accelerometer Hub : Subsystem
  Barometer : Subsystem
  Constant : Constant  Value=8191
  Data Type Conversion6 : DataTypeConversion  OutDataTypeStr=uint32  SaturateOnIntegerOverflow=off  RndMeth=Floor
  Demux : Demux  Outputs=3
  Demux1 : Demux  Outputs=3
  Demux2 : Demux  Outputs=3
  Demux3 : Demux  Outputs=13
  GPS : Subsystem
  Gyroscope Hub : Subsystem
  Magnetometer Hub : Subsystem
  Terminator : Terminator
  Terminator2 : Terminator
  Out Bus Element : Outport  VectorParamsAs1DForOutWhenUnconnected=off  PortName=SensorData  Element=xacc
  Out Bus Element1 : Outport  VectorParamsAs1DForOutWhenUnconnected=off  PortName=SensorData  Element=yacc
  Out Bus Element2 : Outport  VectorParamsAs1DForOutWhenUnconnected=off  PortName=SensorData  Element=zacc
  Out Bus Element3 : Outport  VectorParamsAs1DForOutWhenUnconnected=off  PortName=SensorData  Element=xgyro
  Out Bus Element4 : Outport  VectorParamsAs1DForOutWhenUnconnected=off  PortName=SensorData  Element=ygyro
  Out Bus Element5 : Outport  VectorParamsAs1DForOutWhenUnconnected=off  PortName=SensorData  Element=zgyro
  Out Bus Element6 : Outport  VectorParamsAs1DForOutWhenUnconnected=off  PortName=SensorData  Element=xmag
  Out Bus Element7 : Outport  VectorParamsAs1DForOutWhenUnconnected=off  PortName=SensorData  Element=ymag
  Out Bus Element8 : Outport  VectorParamsAs1DForOutWhenUnconnected=off  PortName=SensorData  Element=zmag
  Out Bus Element9 : Outport  VectorParamsAs1DForOutWhenUnconnected=off  PortName=SensorData  Element=abs_pressure
  Out Bus Element10 : Outport  VectorParamsAs1DForOutWhenUnconnected=off  PortName=SensorData  Element=diff_pressure
  Out Bus Element11 : Outport  VectorParamsAs1DForOutWhenUnconnected=off  PortName=SensorData  Element=pressure_alt
  Out Bus Element12 : Outport  VectorParamsAs1DForOutWhenUnconnected=off  PortName=SensorData  Element=temperature
  Out Bus Element13 : Outport  VectorParamsAs1DForOutWhenUnconnected=off  PortName=SensorData  Element=fields_updated
  Out Bus Element14 : Outport  VectorParamsAs1DForOutWhenUnconnected=off  PortName=SensorData  Element=GPS_u
  Out Bus Element15 : Outport  VectorParamsAs1DForOutWhenUnconnected=off  PortName=SensorData  Element=GPS_l
  Out Bus Element16 : Outport  VectorParamsAs1DForOutWhenUnconnected=off  PortName=SensorData  Element=GPS_h
  Out Bus Element17 : Outport  VectorParamsAs1DForOutWhenUnconnected=off  PortName=SensorData  Element=GPS_eph
  Out Bus Element18 : Outport  VectorParamsAs1DForOutWhenUnconnected=off  PortName=SensorData  Element=GPS_epv
  Out Bus Element19 : Outport  VectorParamsAs1DForOutWhenUnconnected=off  PortName=SensorData  Element=GPS_vel
  Out Bus Element20 : Outport  VectorParamsAs1DForOutWhenUnconnected=off  PortName=SensorData  Element=GPS_cog
  Out Bus Element21 : Outport  VectorParamsAs1DForOutWhenUnconnected=off  PortName=SensorData  Element=GPS_vn
  Out Bus Element22 : Outport  VectorParamsAs1DForOutWhenUnconnected=off  PortName=SensorData  Element=GPS_ve
  Out Bus Element23 : Outport  VectorParamsAs1DForOutWhenUnconnected=off  PortName=SensorData  Element=GPS_vd
  Out Bus Element24 : Outport  VectorParamsAs1DForOutWhenUnconnected=off  PortName=SensorData  Element=GPS_fixtype
  Out Bus Element25 : Outport  VectorParamsAs1DForOutWhenUnconnected=off  PortName=SensorData  Element=GPS_satellites_visible
  Out Bus Element26 : Outport  VectorParamsAs1DForOutWhenUnconnected=off  PortName=SensorData  Element=GPS_headVeh
  wires:
  Demux3/13 -> Out Bus Element26/1
  Demux3/12 -> Out Bus Element25/1
  Demux3/11 -> Out Bus Element24/1
  Demux3/10 -> Out Bus Element23/1
  Demux3/9 -> Out Bus Element22/1
  Demux3/8 -> Out Bus Element21/1
  Demux3/7 -> Out Bus Element20/1
  Demux3/6 -> Out Bus Element19/1
  Demux3/5 -> Out Bus Element18/1
  Demux3/4 -> Out Bus Element17/1
  Demux3/3 -> Out Bus Element16/1
  Demux3/2 -> Out Bus Element15/1
  Demux3/1 -> Out Bus Element14/1
  Data Type Conversion6/1 -> Out Bus Element13/1  "fields_updated"
  Constant/1 -> Data Type Conversion6/1
  Barometer/4(temperature) -> Out Bus Element12/1
  Barometer/3(pressure_alt) -> Out Bus Element11/1
  Barometer/2(diff_pressure) -> Out Bus Element10/1
  Barometer/1(Pressure) -> Out Bus Element9/1
  Demux2/3 -> Out Bus Element8/1
  Demux2/2 -> Out Bus Element7/1
  Demux2/1 -> Out Bus Element6/1
  Demux1/3 -> Out Bus Element5/1
  Demux1/2 -> Out Bus Element4/1
  Demux1/1 -> Out Bus Element3/1
  Demux/3 -> Out Bus Element2/1
  Demux/2 -> Out Bus Element1/1
  Demux/1 -> Out Bus Element/1
  GPS/1(GPS) -> Demux3/1
  Magnetometer Hub/1(Mag_means0) -> Demux2/1
  Magnetometer Hub/2(Mag_means1) -> Terminator2/1
  Gyroscope Hub/1(Wmeans0) -> Demux1/1
  Accelerometer Hub/2(Ameans1) -> Terminator/1
  Accelerometer Hub/1(Ameans0) -> Demux/1
  Kinematics 6DOF Bus/1 -> Gyroscope Hub/1(Kinematics 6DOF Bus), Magnetometer Hub/1(Kinematics 6DOF Bus), GPS/1(Kinematics 6DOF Bus), Accelerometer Hub/2(Kinematics 6DOF Bus)
  Environment Model Bus/1 -> Magnetometer Hub/2(Environment Model Bus), Accelerometer Hub/1(Environment Model Bus), Barometer/1(Environment Model Bus)

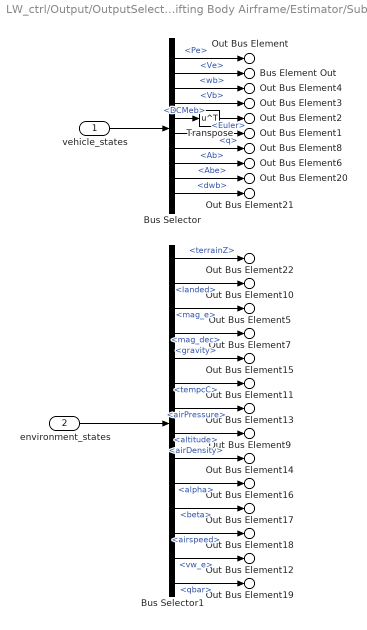
== system LW_ctrl/Output/OutputSelect/Sim/Lifting Body Airframe/Estimator/Subsystem ==
  vehicle_states : Inport
  environment_states : Inport  Port=2
  Bus Selector : BusSelector  OutputSignals=Pe,Ve,wb,Vb,DCMeb,Euler,q,Ab,Abe,dwb
  Bus Selector1 : BusSelector  OutputSignals=terrainZ,landed,mag_e,mag_dec,gravity,tempcC,airPressure,altitude,airDensity,alpha,beta,airspeed,vw_e,qbar
  Transpose : Math  Operator=transpose  SignedPower=on
  Bus Element Out : Outport  PortName=Kinematics 6DOF Bus  Element=Ve
  Out Bus Element : Outport  PortName=Kinematics 6DOF Bus  Element=Xe
  Out Bus Element1 : Outport  PortName=Kinematics 6DOF Bus  Element=Euler
  Out Bus Element2 : Outport  PortName=Kinematics 6DOF Bus  Element=DCM
  Out Bus Element3 : Outport  PortName=Kinematics 6DOF Bus  Element=Vb
  Out Bus Element4 : Outport  PortName=Kinematics 6DOF Bus  Element=Wb
  Out Bus Element6 : Outport  PortName=Kinematics 6DOF Bus  Element=Abb
  Out Bus Element8 : Outport  VectorParamsAs1DForOutWhenUnconnected=off  PortName=Kinematics 6DOF Bus  Element=Quat
  Out Bus Element20 : Outport  PortName=Kinematics 6DOF Bus  Element=Abe
  Out Bus Element21 : Outport  PortName=Kinematics 6DOF Bus  Element=dWb
  Out Bus Element5 : Outport  Port=2  PortName=Environment Model Bus  Element=mag_e
  Out Bus Element7 : Outport  Port=2  PortName=Environment Model Bus  Element=mag_dec
  Out Bus Element9 : Outport  Port=2  PortName=Environment Model Bus  Element=Altitude
  Out Bus Element10 : Outport  Port=2  PortName=Environment Model Bus  Element=landed
  Out Bus Element11 : Outport  Port=2  PortName=Environment Model Bus  Element=TempC
  Out Bus Element12 : Outport  Port=2  PortName=Environment Model Bus  Element=Vwg
  Out Bus Element13 : Outport  Port=2  PortName=Environment Model Bus  Element=AirPressure
  Out Bus Element14 : Outport  Port=2  PortName=Environment Model Bus  Element=Rho
  Out Bus Element15 : Outport  Port=2  PortName=Environment Model Bus  Element=g
  Out Bus Element16 : Outport  Port=2  PortName=Environment Model Bus  Element=alpha
  Out Bus Element17 : Outport  Port=2  PortName=Environment Model Bus  Element=beta
  Out Bus Element18 : Outport  Port=2  PortName=Environment Model Bus  Element=airspeed
  Out Bus Element19 : Outport  Port=2  PortName=Environment Model Bus  Element=qbar
  Out Bus Element22 : Outport  Port=2  PortName=Environment Model Bus  Element=TerrainZ
  wires:
  Transpose/1 -> Out Bus Element2/1
  Bus Selector1/1 -> Out Bus Element22/1  "<terrainZ>"
  Bus Selector/10 -> Out Bus Element21/1  "<dwb>"
  Bus Selector/9 -> Out Bus Element20/1  "<Abe>"
  Bus Selector1/14 -> Out Bus Element19/1  "<qbar>"
  Bus Selector1/13 -> Out Bus Element12/1  "<vw_e>"
  Bus Selector1/12 -> Out Bus Element18/1  "<airspeed>"
  Bus Selector1/11 -> Out Bus Element17/1  "<beta>"
  Bus Selector1/10 -> Out Bus Element16/1  "<alpha>"
  Bus Selector1/9 -> Out Bus Element14/1  "<airDensity>"
  Bus Selector1/8 -> Out Bus Element9/1  "<altitude>"
  Bus Selector1/6 -> Out Bus Element11/1  "<tempcC>"
  Bus Selector1/7 -> Out Bus Element13/1  "<airPressure>"
  Bus Selector1/5 -> Out Bus Element15/1  "<gravity>"
  Bus Selector1/4 -> Out Bus Element7/1  "<mag_dec>"
  Bus Selector1/3 -> Out Bus Element5/1  "<mag_e>"
  Bus Selector1/2 -> Out Bus Element10/1  "<landed>"
  environment_states/1 -> Bus Selector1/1
  Bus Selector/8 -> Out Bus Element6/1  "<Ab>"
  Bus Selector/7 -> Out Bus Element8/1  "<q>"
  Bus Selector/6 -> Out Bus Element1/1  "<Euler>"
  Bus Selector/5 -> Transpose/1  "<DCMeb>"
  Bus Selector/4 -> Out Bus Element3/1  "<Vb>"
  Bus Selector/3 -> Out Bus Element4/1  "<wb>"
  Bus Selector/2 -> Bus Element Out/1  "<Ve>"
  Bus Selector/1 -> Out Bus Element/1  "<Pe>"
  vehicle_states/1 -> Bus Selector/1

== system LW_ctrl/Output/OutputSelect/Sim/Lifting Body Airframe/Estimator/Subsystem2 ==
  In Bus Element1 : Inport  PortName=SensorData  Element=xgyro
  In Bus Element2 : Inport  PortName=SensorData  Element=ygyro
  In Bus Element3 : Inport  PortName=SensorData  Element=zgyro
  In Bus Element4 : Inport  PortName=SensorData  Element=xacc
  In Bus Element5 : Inport  PortName=SensorData  Element=yacc
  In Bus Element6 : Inport  PortName=SensorData  Element=zacc
  Data Type Conversion : DataTypeConversion  OutDataTypeStr=single  SaturateOnIntegerOverflow=off  RndMeth=Floor
  Mux : Mux  Inputs=6
  imu : Outport
  wires:
  In Bus Element3/1 -> Mux/3
  In Bus Element2/1 -> Mux/2
  In Bus Element1/1 -> Mux/1
  In Bus Element4/1 -> Mux/4
  In Bus Element5/1 -> Mux/5
  In Bus Element6/1 -> Mux/6
  Data Type Conversion/1 -> imu/1
  Mux/1 -> Data Type Conversion/1
